simulink model "MesuresAuto_Gauche"  (R2015a)
settings: Solver=FixedStepDiscrete  StartTime=0.0  StopTime=10  FixedStep=Ts_Auto  RelTol=1e-3
values from neighbouring files (symbols this model uses):
  alpha = 10*indice    [MesuresAuto.m]
libraries: Wheels x1
settings Model: SimulationMode=external  ExtModeTrigDuration=2  Creator=tbaroche  LastModifiedBy=tbaroche
settings DataIOCC: LimitDataPoints=off  MaxDataPoints=10000  SaveOutput=off  SaveTime=off
settings OptimizationCC: OptimizeModelRefInitCode=on  LifeSpan=1
settings DebuggingCC: UnderspecifiedInitializationDetection=Classic  MergeDetectMultiDrivingBlocksExec=none
settings HardwareCC: ProdLargestAtomicInteger=Long  ProdLargestAtomicFloat=Double  ProdEndianess=LittleEndian  ProdHWDeviceType=ARM Compatible->ARM Cortex
settings RTWCC: SystemTargetFile=realtime.tlc  GenerateMakefile=off  TemplateMakefile=realtime.tmf  Description=Run on Target Hardware  RTWVerbose=off
settings ERTTargetCC: CombineOutputUpdateFcns=off  ExtModeTransport=3  ExtModeMexFile=ext_serial_win32_comm_rtt  ExtModeMexArgs=0 1 9600  ERTSrcFileBannerTemplate=realtime_code_template.cgt  ERTHdrFileBannerTemplate=realtime_code_template.cgt  ERTDataSrcFileTemplate=realtime_code_template.cgt  ERTDataHdrFileTemplate=realtime_code_template.cgt  ERTCustomFileTemplate=realtime_file_process.tlc

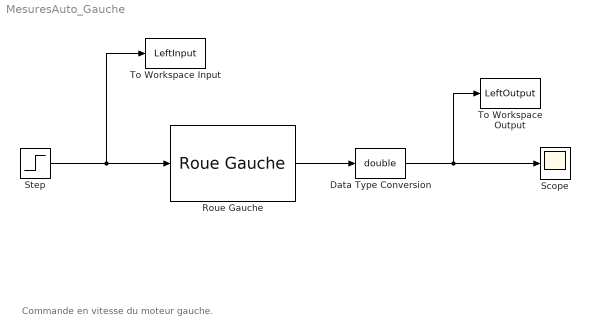
== system MesuresAuto_Gauche ==
  note: Commande en vitesse du moteur gauche.
  Data Type Conversion : DataTypeConversion  OutDataTypeStr=double
  Roue Gauche : Wheels/Roue Gauche
  Scope : Scope
  Step : Step  Time=3  After=alpha  SampleTime=0
  To Workspace Input : ToWorkspace  VariableName=LeftInput  SaveFormat=Structure With Time  SampleTime=-1
  To Workspace Output : ToWorkspace  VariableName=LeftOutput  SaveFormat=Structure With Time  SampleTime=-1
  wires:
  Roue Gauche/1 -> Data Type Conversion/1
  Step/1 -> Roue Gauche/1, To Workspace Input/1
  Data Type Conversion/1 -> To Workspace Output/1, Scope/1
